simulink model "FOC_ctrl"  (R2025b)
settings: Solver=FixedStepAuto  StartTime=0.0  StopTime=Tstop  FixedStep=p.FastTs  RelTol=1e-3
undefined symbols (not defined in the file): angleDeg, c, Inverter, m, Motor, p, torqueNm, Tstop, we
libraries: simulink x5, fl_lib x4, nesl_utility x3, dspsigops x2, ee_lib x1
(part 3 of 3)

== matlab function FOC_ctrl/Clarke-Park-InvPark-InvClarke/State Observer+PLL/PLL/ss_theta_step ==
  data: theta_prev input; we input; Ts input; theta_next output
function theta_next = ss_theta_step(theta_prev, we, Ts)
%SS_THETA_STEP Open-loop electrical angle generator (bench-test stand-in
% for the sensorless STO-PLL observer, sto_pll_speed_pos_fdbk.c, which
% isn't wired into this testbed). Integrates a commanded electrical speed
% `we` [rad/s] once per PWM period and wraps to (-pi, pi], exactly the
% "forced angle" mode used to bring up a current loop before closing the
% speed/position loop on a real drive.
%
% theta_prev : previous period's angle (radians) - feed from a Unit Delay
%              (Z^-1), initial condition 0, same as IaEst/IbEst/IcEst
% we         : commanded electrical speed, rad/s (2*pi*fe)
% Ts         : p.Ts (must match the model's execution rate)

theta_next = theta_prev + we * Ts;
theta_next = mod(theta_next + pi, 2*pi) - pi;

end

== matlab function FOC_ctrl/Clarke-Park-InvPark-InvClarke/SpeedLoop/Speed controller ==
  data: error input; Iq_raw output; IqIntegral_prev input; Kp input; Ki input; KpDiv input; KiDiv input; OutUpper input; OutLower input; IntegUpper input; IntegLower input; IqIntegral_next output
function [Iq_raw, IqIntegral_next] = ss_pi_Speedcontroller(error, IqIntegral_prev, ...
    Kp, Ki, KpDiv, KiDiv, OutUpper, OutLower, IntegUpper, IntegLower)
%SS_PI_CONTROLLER MATLAB port of PI_Controller()
% (MCSDK_v6.4.2-Full/MotorControl/MCSDK/MCLib/Any/Src/pid_regulator.c,
% ~lines 622-738). Used for both the Id and Iq current loops (same
% function, different gains - matches how the firmware reuses one
% PI_Controller() for pPIDId[M1] and pPIDIq[M1]).
%
% Structure: proportional term, integral term (accumulated then clamped
% to [IntegLower,IntegUpper] BEFORE being added to the proportional
% term), summed and clamped to [OutLower,OutUpper] - then, distinctively,
% whatever amount was clamped off ("discharge") is fed back and added to
% the stored integral term. That's back-calculation anti-windup: it stops
% the integrator winding up further while the Iq_raw is saturated,
% without needing a separate windup-detection flag.
%
% NOT ported: the C code's wIntegral_sum_temp int32-overflow guards
% (lines ~654-689) - those exist to protect a 32-bit fixed-point
% accumulator from wrapping around, which isn't a concern in double-
% precision floating point. The control algorithm itself (this function)
% is unaffected by omitting them.
%
% IqIntegral_prev/IqIntegral_next : the PI's stored integral state
% (pHandle->wIntegralTerm) - feed back through a Unit Delay (Z^-1),
% initial condition 0, same pattern as IaEst/IbEst/IcEst and theta_prev
% elsewhere in this build.
%
% error : reference - measured, in the SAME units the gains were tuned
%         for - i.e. raw ADC-digit-equivalent current, NOT Amps (see
%         ss_params.m's "Current-loop PI gains" section for the Amps<->
%         digit and per-unit-voltage<->raw conversions to do at the call
%         site).
% Kp, Ki, KpDiv, KiDiv, OutUpper, OutLower, IntegUpper, IntegLower :
%         p.IQ_* / p.ID_* / p.PI_* from ss_params.m

propTerm = Kp * error;

if Ki == 0
    integralTerm = 0;
else
    integralSum = IqIntegral_prev + Ki * error;
    if integralSum > IntegUpper
        integralTerm = IntegUpper;
    elseif integralSum < IntegLower
        integralTerm = IntegLower;
    else
        integralTerm = integralSum;
    end
end

Iq_raw_raw = propTerm / KpDiv + integralTerm / KiDiv;

discharge = 0;
if Iq_raw_raw > OutUpper
    discharge = OutUpper - Iq_raw_raw;
    Iq_raw = OutUpper;
elseif Iq_raw_raw < OutLower
    discharge = OutLower - Iq_raw_raw;
    Iq_raw = OutLower;
else
    Iq_raw = Iq_raw_raw;
end

IqIntegral_next = integralTerm + discharge * KiDiv;

end

== matlab function FOC_ctrl/compressorLoadProfile/MATLAB Function1 ==
  data: theta_mech_prev input; theta_mech_next output; wmech input; Ts input
function theta_mech_next = ss_mech_angle_step(theta_mech_prev, wmech, Ts)
%SS_MECH_ANGLE_STEP Integrates the rotor/crankshaft's absolute MECHANICAL
% angle (wrapped [0, 2*pi) - one full mechanical revolution). NOT the
% same as ss_theta_step.m's electrical angle, which wraps
% p.MotorPolePairs times faster and loses track of which mechanical
% revolution you're in - needed here because a compressor's load torque
% repeats once per mechanical revolution (crank angle), not once per
% electrical cycle.
%
% theta_mech_prev : previous period's mechanical angle - feed back
%                   through a Unit Delay (Z^-1), initial condition 0
% wmech           : ss_mechanical_model.m's own wmech_next, mechanical
%                   rad/s - UNSCALED (do not multiply by pole_pairs; that
%                   conversion is only for the electrical angle/back-EMF
%                   chain, see ss_theta_step.m / ss_bemf_lookup.m)
% Ts              : p.Ts

theta_mech_next = mod(theta_mech_prev + wmech * Ts, 2*pi);

end

== matlab function FOC_ctrl/compressorLoadProfile/MATLAB Function2 ==
  data: theta_mech input; TL output; angleDeg input; torqueNm input
function TL = ss_load_torque_lookup(theta_mech, angleDeg, torqueNm)
%SS_LOAD_TORQUE_LOOKUP Interpolates the measured load-torque-vs-crank-
% angle table (ss_load_torque_data.m) at the current mechanical angle.
%
% theta_mech : mechanical crank angle, radians, wrapped [0, 2*pi) - feed
%              the DELAYED ss_mech_angle_step.m state (theta_mech_prev),
%              NOT its just-computed theta_mech_next: this value has to
%              be available to compute THIS period's TL feeding
%              ss_mechanical_model.m, which is what produces the speed
%              theta_mech_next is integrated from - using the delayed
%              state avoids a zero-delay algebraic loop, same principle
%              as everywhere else in this build.
% angleDeg, torqueNm : ss_load_torque_data.m output - feed via two
%              Constant blocks (e.g. LoadAngleDeg, LoadTorqueNm), NOT
%              recomputed every step
%
% TL : load torque, Nm, at this instant - feed into
%      ss_mechanical_model.m's TL input (replacing the constant 0.11/0)

theta_deg = mod(theta_mech * 180/pi, 360);
TL = interp1(angleDeg, torqueNm, theta_deg, 'linear');

end

== matlab function FOC_ctrl/Clarke-Park-InvPark-InvClarke/Startup/the phase sequencer ==
  data: t_elapsed input; we_target output; Idref_phase output; Iqref_phase output; phaseNum output; p parameter
function [we_target, Idref_phase, Iqref_phase, phaseNum] = ss_startup_sequencer(t_elapsed, p)
%SS_STARTUP_SEQUENCER MATLAB port of the real startup phase table
% (Inc/drive_parameters.h: PHASE1..5_DURATION / _FINAL_SPEED_UNIT /
% _FINAL_CURRENT_A), the piece that decides what to command DURING
% open-loop alignment + ramp-up, before the sensorless observer is
% trusted (see the OBS_MINIMUM_SPEED_RPM=2400 discussion). This does NOT
% decide which angle to actually use (that's ss_theta_step.m driven by
% we_target here, for phases 1-5) or when/how to hand over to closed-
% loop control (that's the switchover blend, a separate later piece).
%
% Phase table (real firmware values):
%   Phase 1 (align)   : 0.000-0.200 s, hold 0 RPM,      inject 10A on Id
%   Phase 2 (ramp)    : 0.200-0.350 s, ramp to 2500 RPM, inject 10A on Iq
%   Phase 3            : 0.350-0.351 s, ramp to 2510 RPM, 10A on Iq
%   Phase 4            : 0.351-0.352 s, ramp to 2520 RPM, 10A on Iq
%   Phase 5            : 0.352-0.353 s, ramp to 2530 RPM, 10A on Iq
% (Phase 6 - the 25ms TRANSITION_DURATION angle blend - and the switch to
%  the real SpeedLoop's Iqref are separate pieces, not this function.)
%
% Alignment injects along Id (not Iq) because forcing a stator current
% vector at a FIXED, assumed angle only has a stable equilibrium along
% the assumed d-axis - a stator flux there physically attracts the
% rotor's permanent magnet to align with it, which is the whole point of
% this phase (establishing a KNOWN starting position with no feedback
% at all, since back-EMF - and hence any position information - is
% exactly zero at true standstill).
%
% t_elapsed : seconds since the run started - use a Simulink Clock block
%             directly (this whole simulation run IS the startup, so
%             simulation time already starts at 0 - no need for a
%             separate accumulator)
% p         : ss_params() (uses p.MotorPolePairs)
%
% we_target      : commanded electrical speed, rad/s, for
%                  ss_theta_step.m to ramp the FORCED angle toward
%                  during phases 1-5 (this is NOT measured - it's what
%                  a real sensorless drive assumes/forces, since it has
%                  no real angle feedback yet)
% Idref_phase, Iqref_phase : this phase's current references, Amps
% phaseNum       : 1-5 during the sequence, 6 once past phase 5 (ready
%                  for the switchover blend)

% T1 = 0.200; T2 = 0.350; T3 = 0.351; T4 = 0.352; T5 = 0.353; % seconds, cumulative

rpm2we = (2*pi/60) * p.MotorPolePairs;
we_bkpts = p.Startup_RPM * rpm2we;
t_bkpts  = [0, p.Startup_T];

t_clamped = min(t_elapsed, p.Startup_T(end));
we_target = interp1(t_bkpts, we_bkpts, t_clamped, 'linear');

if t_elapsed <= p.Startup_T(1)
    phaseNum = 1;
    Idref_phase = p.Startup_Id_A; Iqref_phase = 0;
elseif t_elapsed <= p.Startup_T(2)
    phaseNum = 2;
    Idref_phase = 0; Iqref_phase = p.Startup_Iq_A;
elseif t_elapsed <= p.Startup_T(3)
    phaseNum = 3;
    Idref_phase = 0; Iqref_phase = p.Startup_Iq_A;
elseif t_elapsed <= p.Startup_T(4)
    phaseNum = 4;
    Idref_phase = 0; Iqref_phase = p.Startup_Iq_A;
elseif t_elapsed <= p.Startup_T(5)
    phaseNum = 5;
    Idref_phase = 0; Iqref_phase = p.Startup_Iq_A;
else
    phaseNum = 6;
    Idref_phase = 0; Iqref_phase = p.Startup_Iq_A; % holds phase-5 values; superseded once the switchover (step 4) hands off
end

end

== matlab function FOC_ctrl/Clarke-Park-InvPark-InvClarke/Iq controller ==
  data: error input; Vq_raw output; IqIntegral_prev input; Kp input; Ki input; KpDiv input; KiDiv input; OutUpper input; OutLower input; IntegUpper input; IntegLower input; IqIntegral_next output
function [Vq_raw, IqIntegral_next] = ss_pi_controllerIq(error, IqIntegral_prev, ...
    Kp, Ki, KpDiv, KiDiv, OutUpper, OutLower, IntegUpper, IntegLower)
%SS_PI_CONTROLLER MATLAB port of PI_Controller()
% (MCSDK_v6.4.2-Full/MotorControl/MCSDK/MCLib/Any/Src/pid_regulator.c,
% ~lines 622-738). Used for both the Id and Iq current loops (same
% function, different gains - matches how the firmware reuses one
% PI_Controller() for pPIDId[M1] and pPIDIq[M1]).
%
% Structure: proportional term, integral term (accumulated then clamped
% to [IntegLower,IntegUpper] BEFORE being added to the proportional
% term), summed and clamped to [OutLower,OutUpper] - then, distinctively,
% whatever amount was clamped off ("discharge") is fed back and added to
% the stored integral term. That's back-calculation anti-windup: it stops
% the integrator winding up further while the Vq_raw is saturated,
% without needing a separate windup-detection flag.
%
% NOT ported: the C code's wIntegral_sum_temp int32-overflow guards
% (lines ~654-689) - those exist to protect a 32-bit fixed-point
% accumulator from wrapping around, which isn't a concern in double-
% precision floating point. The control algorithm itself (this function)
% is unaffected by omitting them.
%
% IqIntegral_prev/IqIntegral_next : the PI's stored integral state
% (pHandle->wIntegralTerm) - feed back through a Unit Delay (Z^-1),
% initial condition 0, same pattern as IaEst/IbEst/IcEst and theta_prev
% elsewhere in this build.
%
% error : reference - measured, in the SAME units the gains were tuned
%         for - i.e. raw ADC-digit-equivalent current, NOT Amps (see
%         ss_params.m's "Current-loop PI gains" section for the Amps<->
%         digit and per-unit-voltage<->raw conversions to do at the call
%         site).
% Kp, Ki, KpDiv, KiDiv, OutUpper, OutLower, IntegUpper, IntegLower :
%         p.IQ_* / p.ID_* / p.PI_* from ss_params.m

propTerm = Kp * error;

if Ki == 0
    integralTerm = 0;
else
    integralSum = IqIntegral_prev + Ki * error;
    if integralSum > IntegUpper
        integralTerm = IntegUpper;
    elseif integralSum < IntegLower
        integralTerm = IntegLower;
    else
        integralTerm = integralSum;
    end
end

Vq_raw_raw = propTerm / KpDiv + integralTerm / KiDiv;

discharge = 0;
if Vq_raw_raw > OutUpper
    discharge = OutUpper - Vq_raw_raw;
    Vq_raw = OutUpper;
elseif Vq_raw_raw < OutLower
    discharge = OutLower - Vq_raw_raw;
    Vq_raw = OutLower;
else
    Vq_raw = Vq_raw_raw;
end

IqIntegral_next = integralTerm + discharge * KiDiv;

end

== matlab function FOC_ctrl/Clarke-Park-InvPark-InvClarke/State Observer+PLL/ss_sto_observer ==
  data: Ialpha_est input; Ialpha_est_next output; Ibeta_est input; Bemf_alpha_est input; Bemf_beta_est input; Ialpha_meas input; Ibeta_meas input; Valpha input; Vbeta input; we_est input; Ibeta_est_next output; Bemf_alpha_est_next output; Bemf_beta_est_next output; p parameter; Ialpha_err output; Ibeta_err output
function [Ialpha_est_next, Ibeta_est_next, Bemf_alpha_est_next, Bemf_beta_est_next, Ialpha_err,Ibeta_err] = ...
    ss_sto_observer_step(Ialpha_est, Ibeta_est, Bemf_alpha_est, Bemf_beta_est, ...
                          Ialpha_meas, Ibeta_meas, Valpha, Vbeta, we_est, p)
%SS_STO_OBSERVER_STEP Stage 1 of the sensorless observer port
% (Src/sto_pll_speed_pos_fdbk.c STO_PLL_CalcElAngle - the Luenberger
% current/back-EMF observer portion only; the PLL angle/speed tracker that
% sits on top of this is a separate, later piece).
%
% This is a MODEL-BASED observer: its prediction step is the exact same
% stator R-L circuit equation as ss_stator_model.m (same Ts, R, L), just
% run in "estimate" space using an ASSUMED/ESTIMATED back-EMF instead of
% the (unknown, to a real sensorless drive) true one. The mismatch between
% the predicted and measured current is the only information available,
% and it's fed back twice:
%   - into the current estimate itself (G1, standard Luenberger correction)
%   - into the back-EMF estimate (G2) - this is what lets the observer
%     actually LEARN the back-EMF rather than just predicting current
%     open-loop from a guessed value
% The back-EMF estimate also carries its own "rotating vector" internal
% model (dEalpha/dt=+we*Ebeta, dEbeta/dt=-we*Ealpha - NOTE the sign: this
% firmware's Clarke transform has a flipped beta axis relative to the
% "textbook" convention, ss_clarke.m's own header - so here
% Ebeta=-Ep*sin(theta) when Ealpha=Ep*cos(theta), which flips the usual
% rotation-coupling sign too. Verified directly: d/dt[Ep*cos(we*t)] =
% -we*Ep*sin(we*t) = +we*Ebeta) - since back-EMF is (to first order) a
% sinusoid at the electrical speed, encoding that rotation directly is
% what lets a CONSTANT pair of gains (G1,G2) track a continuously
% rotating quantity instead of just a fixed one.
%
% Ialpha_est, Ibeta_est, Bemf_alpha_est, Bemf_beta_est : observer state -
%              feed back through four Unit Delay (Z^-1) blocks, initial
%              condition 0 (matches the firmware's own reset value)
% Ialpha_meas, Ibeta_meas : MEASURED stator current, Amps (this build's
%              existing Clarke output - the reconstructed single-shunt
%              current, not a privileged/true value)
% Valpha, Vbeta : ss_rev_park.m output, per-unit (same scale as
%              Va/Vb/Vc/m elsewhere - converted to volts below exactly
%              like ss_stator_model.m does)
% we_est       : estimated electrical speed, rad/s. STAGE 1 VALIDATION
%              ONLY: feed the mechanical model's TRUE we here (there's no
%              PLL yet to produce an estimate) - this is a deliberate,
%              temporary privileged-information shortcut for isolating and
%              validating the observer's own convergence, NOT something to
%              carry into the final startup-sequence integration (that's
%              the exact "true angle for control" trap this build already
%              backed out of once - see ss_angle_blend.m's header). Once
%              Stage 2 (PLL) exists, this input is replaced by the PLL's
%              own output, closing the loop on itself as a real sensorless
%              drive does.
% p            : ss_params() (uses p.MotorRS, p.MotorLS, p.Ts, p.VphaseMax,
%              p.STO_G1, p.STO_G2)
%
% Ialpha_est_next, Ibeta_est_next : updated current estimate, Amps -
%              validate by comparing against the build's own true
%              Ialpha/Ibeta (should track closely, current is measured
%              directly so this is the "easy" half)
% Bemf_alpha_est_next, Bemf_beta_est_next : updated back-EMF estimate,
%              Volts - validate by comparing against Ealpha/Ebeta
%              (ss_clarke.m applied to ss_bemf_lookup.m's output) - THIS
%              is the real test of the observer, since back-EMF is never
%              measured directly, only inferred from the current-error

Valpha_v = Valpha ;
Vbeta_v  = Vbeta  ;

Ialpha_err = Ialpha_est - Ialpha_meas;
Ibeta_err  = Ibeta_est  - Ibeta_meas;

Ialpha_est_next = Ialpha_est + (p.Ts/p.MotorLS)*(Valpha_v - p.MotorRS*Ialpha_est - Bemf_alpha_est) ...
                  + p.STO_G1*Ialpha_err;
Ialpha_est_next = min(max(Ialpha_est_next, -p.MaxReadableCurrent_A), p.MaxReadableCurrent_A);
Ibeta_est_next  = Ibeta_est  + (p.Ts/p.MotorLS)*(Vbeta_v  - p.MotorRS*Ibeta_est  - Bemf_beta_est) ...
                  + p.STO_G1*Ibeta_err;
Ibeta_est_next  = min(max(Ibeta_est_next,  -p.MaxReadableCurrent_A), p.MaxReadableCurrent_A);

Ke =0.00441;         %K_e =0.014954  V/(rad/s) to do
bemfFloorV = 0.2;   % minimum clamp bound, volts — prevents the we_est=0 deadlock
bemfClampBound = max(Ke * abs(we_est) * 3, bemfFloorV);% 3x margin, tune as needed

Bemf_alpha_est_next = Bemf_alpha_est + p.Ts*we_est*Bemf_beta_est  + p.STO_G2*Ialpha_err;
%Bemf_alpha_est_next = min(max(Bemf_alpha_est_next, -p.PLL_BemfPeak_V*1.2), p.PLL_BemfPeak_V*1.2);
%Bemf_alpha_est_next = min(max(Bemf_alpha_est_next, -3.5*1.2), 3.5*1.2);
Bemf_alpha_est_next = min(max(Bemf_alpha_est_next, -bemfClampBound), bemfClampBound);

Bemf_beta_est_next  = Bemf_beta_est  - p.Ts*we_est*Bemf_alpha_est + p.STO_G2*Ibeta_err;
%Bemf_beta_est_next  = min(max(Bemf_beta_est_next,  -p.PLL_BemfPeak_V*1.2), p.PLL_BemfPeak_V*1.2);
%Bemf_beta_est_next  = min(max(Bemf_beta_est_next,  -3.5*1.2), 3.5*1.2);
Bemf_beta_est_next  = min(max(Bemf_beta_est_next,  -bemfClampBound), bemfClampBound);
end

== matlab function FOC_ctrl/Clarke-Park-InvPark-InvClarke/Startup/ reference switcher ==
  data: phaseNum input; Idref output; Idref_phase input; Iqref_phase input; Iqref_speedloop input; Iqref output
function [Idref, Iqref] = ss_startup_ref_switch(phaseNum, Idref_phase, Iqref_phase, Iqref_speedloop)
%SS_STARTUP_REF_SWITCH Selects the Id/Iq current references: the
% open-loop startup sequencer's values during phases 1-5 (alignment +
% forced ramp-up, ss_startup_sequencer.m), or the real closed-loop
% SpeedLoop's output once past phase 5 (phaseNum==6, i.e. during the
% switchover transition and normal running afterward).
%
% phaseNum          : ss_startup_sequencer.m output
% Idref_phase, Iqref_phase : ss_startup_sequencer.m output
% Iqref_speedloop   : the existing SpeedLoop subsystem's Iqref output
%                      (Amps, already rate-transitioned up to p.Ts)
%
% Idref, Iqref : feed these into the existing Id/Iq PI controllers,
%                replacing whatever directly fed Idref_digit/Iqref_digit
%                before (this block now sits between those sources and
%                the PI controllers)

if phaseNum <= 5
    Idref = Idref_phase;
    Iqref = Iqref_phase;
else
    Idref = 0;
    Iqref = Iqref_speedloop;
end

end

== matlab function FOC_ctrl/Clarke-Park-InvPark-InvClarke/Startup/angle blend ==
  data: theta_forced input; theta_used output; theta_real input; t_elapsed input; T5 input; TransitionDuration input; alpha output
function [theta_used, alpha] = ss_angle_blend(theta_forced, theta_real, t_elapsed, T5, TransitionDuration)
%SS_ANGLE_BLEND Selects/blends between the open-loop FORCED angle
% (ss_theta_step.m driven by ss_startup_sequencer.m's we_target) and the
% REAL mechanical angle, matching the real firmware's TRANSITION_DURATION
% (Inc/drive_parameters.h, 25 ms) switchover from forced/assumed
% commutation to the sensorless observer's estimate.
%
% Blending naively (theta_used = (1-alpha)*theta_forced + alpha*theta_real)
% is wrong for angles: they wrap at +-pi, so two angles on opposite sides
% of the wrap boundary (e.g. 3.0 and -3.0, which are almost the same
% physical angle) would blend through completely the wrong side of the
% circle. Standard fix: blend the unit-vector (cos,sin) representation of
% each angle (no discontinuity anywhere) and recover the blended angle via
% atan2 - this always takes the shortest angular path between the two.
%
% t_elapsed  : seconds since the run started (same Clock signal feeding
%              ss_startup_sequencer.m)
% T5         : end of phase 5, seconds (0.353 - matches
%              ss_startup_sequencer.m's T5; pass the same literal or a
%              shared constant so they can't drift apart)
% TransitionDuration : 0.025 (TRANSITION_DURATION, seconds)
%
% theta_used : feed this into Park AND Rev_Park (both must use the SAME
%              angle each period - never mix, or Park/Rev_Park stop being
%              exact inverses of each other, breaking the loop exactly
%              like the algebraic-loop/units bugs earlier in this build)
% alpha      : 0 (pure forced) -> 1 (pure real) - exposed for
%              diagnostics/scoping, not required downstream

alpha = (t_elapsed - T5) / TransitionDuration;
alpha = min(max(alpha, 0), 1);

c = (1-alpha)*cos(theta_forced) + alpha*cos(theta_real);
s = (1-alpha)*sin(theta_forced) + alpha*sin(theta_real);

theta_used = atan2(s, c);

end

== matlab function FOC_ctrl/Clarke-Park-InvPark-InvClarke/State Observer+PLL/ss_speed_filter_step ==
  data: we_est input; we_avg output
function we_avg = ss_speed_filter_step(we_est)
persistent buf idx initialized
N = 128;   % matches ST's STO_FIFO_DEPTH_DPP=32 -> ~2.56ms window at your 12.5kHz rate
if isempty(initialized)
    buf = zeros(1,N);
    idx = 1;
    initialized = true;
end
buf(idx) = we_est;
idx = idx + 1;
if idx > N
    idx = 1;
end
we_avg = sum(buf)/N;

== matlab function FOC_ctrl/Clarke-Park-InvPark-InvClarke/Startup/forced angle generator ==
  data: theta_prev input; theta_forced output; we input; p parameter
function theta_forced  = ss_theta_step(theta_prev, we, p)
%SS_THETA_STEP Open-loop electrical angle generator (bench-test stand-in
% for the sensorless STO-PLL observer, sto_pll_speed_pos_fdbk.c, which
% isn't wired into this testbed). Integrates a commanded electrical speed
% `we` [rad/s] once per PWM period and wraps to (-pi, pi], exactly the
% "forced angle" mode used to bring up a current loop before closing the
% speed/position loop on a real drive.
%
% theta_prev : previous period's angle (radians) - feed from a Unit Delay
%              (Z^-1), initial condition 0, same as IaEst/IbEst/IcEst
% we         : commanded electrical speed, rad/s (2*pi*fe)
% Ts         : p.Ts (must match the model's execution rate)

theta_forced  = theta_prev + we * p.Ts;
theta_forced  = mod(theta_forced  + pi, 2*pi) - pi;

end

== matlab function FOC_ctrl/Clarke-Park-InvPark-InvClarke/calculateAngleError ==
  data: theta_ele input; angErr_deg output; theta_est_next input
function angErr_deg = calculateAngleError(theta_ele,theta_est_next)
%CALCULATEANGLEERROR Computes the wrapped angular error in degrees [-180, 180).
angErr_deg = mod((theta_ele - theta_est_next)*180/pi + 180, 360) - 180;
end

== matlab function FOC_ctrl/Clarke-Park-InvPark-InvClarke/Feed-forward/ss_mech_angle_est ==
  data: theta_mech_est_prev input; theta_mech_est_next output; we_est_mech input; Ts input; alpha input; theta_mech_true input
function theta_mech_est_next = ss_mech_angle_est(theta_mech_est_prev, we_est_mech, Ts, alpha, theta_mech_true)
persistent hasResynced
if isempty(hasResynced)
    hasResynced = false;
end
if ~hasResynced && alpha >= 0.99
    theta_mech_est_next = mod(theta_mech_true, 2*pi);   % one-shot: snap to ground truth right after handoff
    hasResynced = true;
else
    theta_mech_est_next = mod(theta_mech_est_prev + we_est_mech*Ts, 2*pi);  % normal integration otherwise
end

== matlab function FOC_ctrl/Clarke-Park-InvPark-InvClarke/Feed-forward/ss_ff_lookup ==
  data: theta_mech_est input; TL_ff output; angleDeg input; torqueNm input
function TL_ff = ss_ff_lookup(theta_mech_est, angleDeg, torqueNm)
theta_deg = mod(theta_mech_est*180/pi, 360);
TL_ff = interp1(angleDeg, torqueNm, theta_deg, 'linear');
end

== matlab function FOC_ctrl/Clarke-Park-InvPark-InvClarke/compression detection/ss_vmag_compute ==
  data: Valpha input; Vmag output; Vbeta input
function Vmag = ss_vmag_compute(Valpha, Vbeta)
%SS_VMAG_COMPUTE Frame-invariant voltage-command magnitude.
% sqrt(Valpha^2+Vbeta^2) = sqrt(Vd^2+Vq^2) for ANY rotating reference
% frame, so this carries the load-induced slip signature during forced
% startup without needing to know the (assumed, not necessarily correct)
% forced commutation angle.
Vmag = sqrt(Valpha^2 + Vbeta^2);
end

== matlab function FOC_ctrl/Clarke-Park-InvPark-InvClarke/compression detection/ss_tdc_detector_vmag ==
  data: Vmag input; t_elapsed input; MIN_TIME input; MAX_TIME input; we_target input; polePairs input; tdcConfirmed output; candidateTimeOut output; peakVmag output
function [tdcConfirmed, candidateTimeOut, peakVmag] = ss_tdc_detector_vmag_gated(Vmag, t_elapsed, MIN_TIME, MAX_TIME, we_target, polePairs)
%SS_TDC_DETECTOR_VMAG_GATED Local-max detector on |V|, confirmed against
% the KNOWN commanded forced-ramp period (from we_target, the
% controller's own open-loop ramp setpoint) instead of against the
% previous candidate interval. A same-size, ~constant-rate ripple that
% is NOT mechanically locked (its rate does not scale with 60/RPM like
% the real compression event does) will essentially never fall within
% tolerance of the expected revolution period, no matter how self-
% consistent it looks on its own.
persistent Vmag_prev1 Vmag_prev2 recentMin initialized
persistent lastAcceptedTime lastConfirmedTime
if isempty(initialized)
    Vmag_prev1 = 0; Vmag_prev2 = 0; recentMin = 0; initialized = true;
    lastAcceptedTime = -1e9; lastConfirmedTime = -1e9;
end
PROMINENCE_THRESH = 0.15;  % Volts -- real vs ripple can't be told apart
                           % by amplitude alone (confirmed empirically);
                           % this just rejects sub-threshold noise, the
                           % PERIOD_TOL gate below does the real work
PERIOD_TOL = 0.15;         % tightened from an initial 0.40, which still
                           % let some ripple slip through near the window
                           % edge; 0.15 gave a clean 1:1 count match
REFRACTORY = 0.005;

tdcConfirmed = false;
candidateTimeOut = -1;
peakVmag = 0;
inWindow = (t_elapsed >= MIN_TIME) && (t_elapsed <= MAX_TIME);
pastRefractory = (t_elapsed - lastAcceptedTime) >= REFRACTORY;
isLocalMax = inWindow && pastRefractory && (Vmag_prev1 > Vmag_prev2) && (Vmag_prev1 > Vmag) && ((Vmag_prev1 - recentMin) > PROMINENCE_THRESH);

if isLocalMax
    recentMin = Vmag_prev1;
    candidateTime = t_elapsed;
    candidateTimeOut = candidateTime;
    peakVmag = Vmag_prev1;
    lastAcceptedTime = candidateTime;

    we_target_safe = max(we_target, 1e-3);
    expectedPeriod = (2*pi*polePairs) / we_target_safe;

    if lastConfirmedTime <= -1e8
        % bootstrap -- no reference yet. Do NOT emit this as a confirmed
        % detection (it could easily be a ripple candidate); just
        % silently anchor the reference for the next comparison.
        lastConfirmedTime = candidateTime;
    else
        sinceLastConfirmed = candidateTime - lastConfirmedTime;
        if sinceLastConfirmed > 0 && abs(sinceLastConfirmed - expectedPeriod)/expectedPeriod < PERIOD_TOL
            tdcConfirmed = true;
            lastConfirmedTime = candidateTime;
        end
    end
else
    if inWindow && Vmag < recentMin
        recentMin = Vmag;
    end
end
Vmag_prev2 = Vmag_prev1;
Vmag_prev1 = Vmag;
end

== matlab function FOC_ctrl/Clarke-Park-InvPark-InvClarke/Id controller ==
  data: error input; Vd_raw output; IdIntegral_prev input; Kp input; Ki input; KpDiv input; KiDiv input; OutUpper input; OutLower input; IntegUpper input; IntegLower input; IdIntegral_next output
function [Vd_raw, IdIntegral_next] = ss_pi_controllerIq(error, IdIntegral_prev, ...
    Kp, Ki, KpDiv, KiDiv, OutUpper, OutLower, IntegUpper, IntegLower)
%SS_PI_CONTROLLER MATLAB port of PI_Controller()
% (MCSDK_v6.4.2-Full/MotorControl/MCSDK/MCLib/Any/Src/pid_regulator.c,
% ~lines 622-738). Used for both the Id and Iq current loops (same
% function, different gains - matches how the firmware reuses one
% PI_Controller() for pPIDId[M1] and pPIDIq[M1]).
%
% Structure: proportional term, integral term (accumulated then clamped
% to [IntegLower,IntegUpper] BEFORE being added to the proportional
% term), summed and clamped to [OutLower,OutUpper] - then, distinctively,
% whatever amount was clamped off ("discharge") is fed back and added to
% the stored integral term. That's back-calculation anti-windup: it stops
% the integrator winding up further while the Vd_raw is saturated,
% without needing a separate windup-detection flag.
%
% NOT ported: the C code's wIntegral_sum_temp int32-overflow guards
% (lines ~654-689) - those exist to protect a 32-bit fixed-point
% accumulator from wrapping around, which isn't a concern in double-
% precision floating point. The control algorithm itself (this function)
% is unaffected by omitting them.
%
% IdIntegral_prev/IdIntegral_next : the PI's stored integral state
% (pHandle->wIntegralTerm) - feed back through a Unit Delay (Z^-1),
% initial condition 0, same pattern as IaEst/IbEst/IcEst and theta_prev
% elsewhere in this build.
%
% error : reference - measured, in the SAME units the gains were tuned
%         for - i.e. raw ADC-digit-equivalent current, NOT Amps (see
%         ss_params.m's "Current-loop PI gains" section for the Amps<->
%         digit and per-unit-voltage<->raw conversions to do at the call
%         site).
% Kp, Ki, KpDiv, KiDiv, OutUpper, OutLower, IntegUpper, IntegLower :
%         p.IQ_* / p.ID_* / p.PI_* from ss_params.m

propTerm = Kp * error;

if Ki == 0
    integralTerm = 0;
else
    integralSum = IdIntegral_prev + Ki * error;
    if integralSum > IntegUpper
        integralTerm = IntegUpper;
    elseif integralSum < IntegLower
        integralTerm = IntegLower;
    else
        integralTerm = integralSum;
    end
end

Vd_raw_raw = propTerm / KpDiv + integralTerm / KiDiv;

discharge = 0;
if Vd_raw_raw > OutUpper
    discharge = OutUpper - Vd_raw_raw;
    Vd_raw = OutUpper;
elseif Vd_raw_raw < OutLower
    discharge = OutLower - Vd_raw_raw;
    Vd_raw = OutLower;
else
    Vd_raw = Vd_raw_raw;
end

IdIntegral_next = integralTerm + discharge * KiDiv;

end

== matlab function FOC_ctrl/PWM_PhaseCurrent/SVPWM_minmax ==
  data: Va input; dA output; Vb input; Vc input; dB output; dC output
function [dA, dB, dC] = ss_svpwm_minmax(Va, Vb, Vc)
%SS_SVPWM_MINMAX Carrier-based SVPWM via min-max common-mode injection.
%
% Standard trick to get space-vector-equivalent modulation without ever
% computing a vector angle or sector: subtract the average of the largest
% and smallest of the three instantaneous reference voltages from all
% three. That "third-harmonic-like" zero-sequence term cancels line-to-
% line (so it doesn't affect the actual motor voltages) but centers the
% three duty cycles inside the 0..1 carrier range, extending the linear
% modulation range from m=1 (plain sine-triangle) to m=2/sqrt(3)~=1.1547
% (six-step limit) - the same range single-shunt SVPWM assumes.
%
% This is the same formula used inline in
% test_single_shunt_reconstruction.m (and export_for_simulink.m); pulled
% out here so it can be dropped into a Simulink MATLAB Function block and
% reused instead of duplicated.
%
% Va, Vb, Vc : per-unit reference phase voltages, nominally in [-1, 1]
%              (e.g. Va = m*cos(theta_e), 120 deg apart), where m is the
%              modulation index.
%
% dA, dB, dC : duty cycle in [0, 1], ready for the next stage (converting
%              to timer counter/CCR values, i.e. CntPhX = round(dX *
%              Half_PWMPeriod) - NOT done here on purpose, kept as a
%              separate step).

v0 = -(max([Va, Vb, Vc]) + min([Va, Vb, Vc])) / 2;

dA = 0.5 + 0.5 * (Va + v0);
dB = 0.5 + 0.5 * (Vb + v0);
dC = 0.5 + 0.5 * (Vc + v0);

end

== matlab function FOC_ctrl/PWM_PhaseCurrent/sector_from_duty ==
  data: dA input; lowDuty output; dB input; dC input; midDuty output; highDuty output; sector output
function [lowDuty, midDuty, highDuty, sector] = ss_sector_from_duty(dA, dB, dC)
%SS_SECTOR_FROM_DUTY Single-shunt "sector" (1-6) from the ranking of the
% three phase duty cycles, plus the low/mid/high phase-index table used by
% the firmware's SingleShuntTopology branch.
%
% Source: Src/pwm_curr_fdbk.c, PWMC_SetPhaseVoltage() (~lines 190-320).
% For SingleShuntTopology==true, ST hard-codes lowDuty/midDuty/highDuty
% per sector instead of sorting the duty values at runtime:
%
%   SECTOR_1: low=C(2) mid=B(1) high=A(0)
%   SECTOR_2: low=C(2) mid=A(0) high=B(1)
%   SECTOR_3: low=A(0) mid=C(2) high=B(1)
%   SECTOR_4: low=A(0) mid=B(1) high=C(2)
%   SECTOR_5: low=B(1) mid=A(0) high=C(2)
%   SECTOR_6: low=B(1) mid=C(2) high=A(0)
%
% Those 6 fixed tables are simply the 6 possible strict orderings of
% (A,B,C) duty - which is exactly what single-shunt sampling cares about,
% since it is the ORDER the three legs switch in (not the SVM angle
% itself) that determines which phase current flows through the shunt
% during each sub-interval. Ranking the actual duty values here is
% therefore equivalent to, but independent of, ST's fixed-point angle
% (wX/wY/wZ) sector computation - it removes any risk of an angle-
% convention mismatch while producing identical low/mid/high results for
% any physically valid duty pattern.
%
% dA, dB, dC : commanded ON-time duty of phase A/B/C, any consistent unit
%              (ticks or 0..1), this period.
%
% Returns 0-based phase indices (0=A, 1=B, 2=C) for lowDuty/midDuty/highDuty,
% matching pHandle->lowDuty/midDuty/highDuty in the C driver.

d = [dA, dB, dC];
[~, order] = sort(d);              % order(1) = index(1-based) of smallest duty
low  = order(1) - 1;
mid  = order(2) - 1;
high = order(3) - 1;

table = [ 2 1 0;   % SECTOR_1
          2 0 1;   % SECTOR_2
          0 2 1;   % SECTOR_3
          0 1 2;   % SECTOR_4
          1 0 2;   % SECTOR_5
          1 2 0 ]; % SECTOR_6

idx = find(all(table == [low mid high], 2), 1);
if ~isempty(idx)
    sector = idx(1);
else
    sector = 1; % or handle error / default case
end
lowDuty = low;
midDuty = mid;
highDuty = high;
end

== matlab function FOC_ctrl/PWM_PhaseCurrent/calc_duty_and_samplepoints ==
  data: CntPhA input; DmaBuffCCR_up output; CntPhB input; CntPhC input; lowDuty input; midDuty input; highDuty input; DmaBuffCCR_down output; SamplePoint1 output; SamplePoint2 output; iflag output; p parameter
function [DmaBuffCCR_up, DmaBuffCCR_down, SamplePoint1, SamplePoint2, iflag] = ...
    ss_calc_duty_and_samplepoints(CntPhA, CntPhB, CntPhC, lowDuty, midDuty, highDuty, p)
%SS_CALC_DUTY_AND_SAMPLEPOINTS MATLAB port of R1_CalcDutyCycles()
% (Src/r1_ps_pwm_curr_fdbk.c, ~lines 1097-1282).
%
% Every PWM period, single-shunt sensing needs two ADC injected
% conversions of the DC-link shunt current, timed to fall inside the two
% "two-phases-on" sub-intervals either side of the mid-duty phase's
% switching edges. Those windows only exist, and are only wide enough to
% trigger + finish a conversion (>= p.TMin ticks), when the three duty
% cycles are far enough apart. Close to a sector boundary (two duties
% nearly equal) the natural window collapses, so this function:
%
%   1) checks the two natural gaps (high-mid, mid-low) against TMin;
%   2) if a gap is too small but can still be opened by shifting the
%      shorter leg's compare value by a few ticks, does so via aShiftval
%      (kept symmetric: +shift in the first half of the center-aligned
%      PWM period, -shift in the second half, so the AVERAGE duty over
%      the full period - and thus the commanded voltage - is unchanged);
%   3) if even that isn't possible (duty pinned near 0% or 100%), marks
%      that phase as unavailable this period (iflag bit cleared) and
%      falls back to one fixed sampling point at mid-period;
%   4) returns iflag (IA_OK/IB_OK/IC_OK bits) telling
%      ss_get_phase_currents() which phase current(s) can be trusted from
%      this period's two ADC samples, and which must fall back to an
%      estimate instead.
%
% Inputs are all timer ticks (see ss_params, matches p.HalfPwmPeriod).
% CntPhA/B/C : commanded compare values (0..p.HalfPwmPeriod)
% lowDuty/midDuty/highDuty : 0-based phase index (0=A,1=B,2=C), from
%                            ss_sector_from_duty
%
% Outputs:
% DmaBuffCCR_up/down : shifted CCR values for the up-count / down-count
%                      half of the period (mirrors DmaBuffCCR[0:2] and
%                      DmaBuffCCR[4:6])
% SamplePoint1/2     : ADC trigger points in timer ticks (TIM1_CH5/CH6)
% iflag              : uint8 bitmask, bit0=IA_OK bit1=IB_OK bit2=IC_OK

IA_OK = uint8(1); IB_OK = uint8(2); IC_OK = uint8(4);
ALFLAG = [IA_OK IB_OK IC_OK];

aCCRval = [CntPhA, CntPhB, CntPhC];
maxVal = highDuty + 1;   % to 1-based MATLAB index
midIdx = midDuty  + 1;
minVal = lowDuty  + 1;

iflag = uint8(0);
aShiftval = [0 0 0];

submax_mid          = aCCRval(maxVal) - aCCRval(midIdx);
submax_mid_deltmin   = submax_mid - p.TMin;
submid_min           = aCCRval(midIdx) - aCCRval(minVal);
submid_min_deltmin   = submid_min - p.TMin;
max_bad_flag = false;
min_bad_flag = false;

if submax_mid_deltmin > 0
    iflag = bitor(iflag, ALFLAG(maxVal));
else
    if (1 - submax_mid_deltmin + aCCRval(maxVal) + p.hTADConv) > p.HalfPwmPeriod
        max_bad_flag = true;            % no room to open a window even after shifting
    else
        iflag = bitor(iflag, ALFLAG(maxVal));
        aShiftval(maxVal) = 1 - submax_mid_deltmin;
    end
end

if submid_min_deltmin > 0
    iflag = bitor(iflag, ALFLAG(minVal));
else
    if (submid_min_deltmin - 1 + aCCRval(minVal)) < 0
        min_bad_flag = true;
    else
        iflag = bitor(iflag, ALFLAG(minVal));
        aShiftval(minVal) = submid_min_deltmin - 1;
    end
end

if (~max_bad_flag) && (~min_bad_flag)
    SamplePoint1 = aCCRval(midIdx) - p.TSample;
    SamplePoint2 = aCCRval(midIdx) + p.TMin - p.TSample;
elseif max_bad_flag && min_bad_flag
    SamplePoint1 = p.HalfPwmPeriod / 2;
    SamplePoint2 = SamplePoint1 + p.TSample + p.hTADConv;
elseif max_bad_flag
    SamplePoint1 = aCCRval(midIdx) - p.TSample;
    SamplePoint2 = aCCRval(midIdx) + p.hTADConv;
else
    SamplePoint2 = aCCRval(midIdx) + p.TMin - p.TSample;
    SamplePoint1 = aCCRval(midIdx);
end


if (SamplePoint2 - SamplePoint1) < p.hTADConv
    iflag = bitand(iflag, ALFLAG(maxVal));
    iflag = bitand(iflag, bitcmp(ALFLAG(minVal)));
    SamplePoint1 = p.HalfPwmPeriod / 2;
    SamplePoint2 = SamplePoint1 + p.TSample + p.hTADConv;
end

if (SamplePoint2 >= p.HalfPwmPeriod) || (SamplePoint2 <= 0)
    iflag = bitand(iflag, ALFLAG(maxVal));
    SamplePoint2 = aCCRval(midIdx) + p.hTADConv;
end
if (SamplePoint1 >= p.HalfPwmPeriod) || (SamplePoint1 <= 0)
    iflag = bitand(iflag, bitcmp(ALFLAG(minVal)));
    SamplePoint1 = aCCRval(midIdx);
end

DmaBuffCCR_up   = [CntPhA, CntPhB, CntPhC] + aShiftval;   % up-count half   (DmaBuffCCR[0:2])
DmaBuffCCR_down = [CntPhA, CntPhB, CntPhC] - aShiftval;   % down-count half (DmaBuffCCR[4:6])

end
